simulink library "makeOcT_cl"  (R2020a)
settings: Solver=VariableStepAuto  StartTime=0.0  StopTime=10.0  RelTol=1e-3
libraries: rotationAboutY x1, rotationAboutZ x1
settings Model: Creator=Ayaz  LastModifiedBy=Ayaz

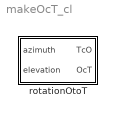
== system makeOcT_cl ==
  rotationOtoT : Subsystem

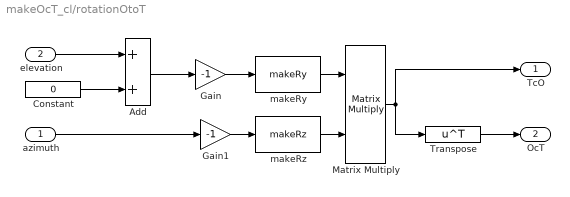
== system makeOcT_cl/rotationOtoT ==
  azimuth : Inport
  elevation : Inport  Port=2
  Add : Sum
  Constant : Constant  Value=0
  Gain : Gain  Gain=-1
  Gain1 : Gain  Gain=-1
  Matrix Multiply : Product  Multiplication=Matrix(*)
  Transpose : Math  Operator=transpose  SaturateOnIntegerOverflow=on
  makeRy : rotationAboutY/makeRy  SystemSampleTime=-1  Latency=0  AutoFrameSizeCalculation=off
  makeRz : rotationAboutZ/makeRz  SystemSampleTime=-1  Latency=0  AutoFrameSizeCalculation=off
  TcO : Outport
  OcT : Outport  Port=2
  wires:
  Gain/1 -> makeRy/1
  Matrix Multiply/1 -> TcO/1, Transpose/1
  azimuth/1 -> Gain1/1
  makeRz/1 -> Matrix Multiply/2
  Transpose/1 -> OcT/1
  elevation/1 -> Add/1
  Constant/1 -> Add/2
  Add/1 -> Gain/1
  makeRy/1 -> Matrix Multiply/1
  Gain1/1 -> makeRz/1
